simulink model "IEEE24bus"  (R2019b)
settings: Solver=VariableStepAuto  StartTime=0.0  StopTime=100  RelTol=1e-3
values from neighbouring files (symbols this model uses):
  C_b = 1/(w_b*Z_b)    (= 5.01433343075e-06)    [IEEE24_bus.m]
  Exc = [ 011	0	 200	0.02	1.12   0.5   0	0       0       0       0       0 ... (first row only)    [IEEE24_bus.m]
  G_data = [ 011	15.8 138	2.8	0.2     2.7	1.5     0.3     7.5     0.25	0.04	0.85	0.85	0.25	0.12	0 ... (first row only)    [IEEE24_bus.m]
  H011 = 4    [IEEE24_bus.m]
  H012 = 4    [IEEE24_bus.m]
  H013 = 4    [IEEE24_bus.m]
  H021 = 4    [IEEE24_bus.m]
  H022 = 4    [IEEE24_bus.m]
  H023 = 4    [IEEE24_bus.m]
  H024 = 4    [IEEE24_bus.m]
  H025 = 4    [IEEE24_bus.m]
  H026 = 4    [IEEE24_bus.m]
  H131 = 4    [IEEE24_bus.m]
  H132 = 4    [IEEE24_bus.m]
  H133 = 4    [IEEE24_bus.m]
  H134 = 4    [IEEE24_bus.m]
  H135 = 4    [IEEE24_bus.m]
  H151 = 4    [IEEE24_bus.m]
  H152 = 4    [IEEE24_bus.m]
  H153 = 4    [IEEE24_bus.m]
  H154 = 4    [IEEE24_bus.m]
  H161 = 4    [IEEE24_bus.m]
  H181 = 3.25    [IEEE24_bus.m]
  H211 = 4    [IEEE24_bus.m]
  H212 = 4    [IEEE24_bus.m]
  H213 = 4    [IEEE24_bus.m]
  H215 = 4    [IEEE24_bus.m]
  H216 = 4    [IEEE24_bus.m]
  H221 = 3.25    [IEEE24_bus.m]
  H231 = 4    [IEEE24_bus.m]
  H232 = 4    [IEEE24_bus.m]
  H233 = 4    [IEEE24_bus.m]
  H234 = 4    [IEEE24_bus.m]
  H235 = 4    [IEEE24_bus.m]
  L_b = Z_b/w_b    (= 1.40321608159)    [IEEE24_bus.m]
  PSSMODEL = 1    [IEEE24_bus.m]    (also in IEEE24bus_simplified_benchmark.m)
  Z_b = (V_b^2)/S_b    (= 529)    [IEEE24_bus.m]
undefined symbols (not defined in the file or in its folder): D1, Delta
libraries: powerlib x258, sps_avr x33, microgridLibrary x6
(part 5 of 6)

== system IEEE24bus/212 ==
  212 : powerlib/Machines/Synchronous Machine pu Standard  PresetModel=No  MechanicalLoad=Mechanical power Pm  ShowDetailedParameters=on  RotorType=Round  Units=per unit standard parameters  MeasurementBus=off  NominalParameters="[120*1E6  G_data(24,3)*1E3  60]"  Reactances1=[G_data(24,6),G_data(24,8),G_data(24,10),G_data(24,7),G_data(24,12),G_data(24,14),G_data(24,5)]  Reactances2=[G_data(6,6),G_data(6,8),G_data(6,10),G_data(6,7),G_data(6,12),G_data(6,14),G_data(6,5)]  dAxisTimeConstants=Open-circuit  qAxisTimeConstants=Open-circuit  TimeConstants1="[G_data(6,9)  G_data(6,11)  G_data(6,13)  G_data(6,15)]"  TimeConstants2="[G_data(24,9)  G_data(24,11)  G_data(24,13)  G_data(24,15)]"  TimeConstants3="[  5.9  0.033  0.023  ]"  TimeConstants4=[ 8.0, 0.03, 0.3371, 0.0295 ]  TimeConstants5=[ 1.01, 0.053, 0.1 ]  TimeConstants6=[ 1.3201, 0.023, 1.0, 0.07 ]  TimeConstants7="[  1.01  0.053  0.051266  ]"  TimeConstants8=[ 1.3201, 0.0231, 0.3371, 0.0295 ]  StatorResistance=0  Mechanical="[ H212 0  4 ]"  PolePairs=4  InitialConditions=[0 -49.0871 0.832503 0.832503 0.832503 -10.6328 -130.633 109.367 2.39024]  SetSaturation=off  Saturation=[0.6404,0.7127,0.8441,0.9214,0.9956,1.082,1.19,1.316,1.457;0.7,0.7698,0.8872,0.9466,0.9969,1.046,1.1,1.151,1.201]  LoadFlowParameters=[1 3330000000 20000 0 0]  TsPowergui=0  TsBlock=-1  IterativeModel=Forward Euler  IterativeDiscreteModel=Trapezoidal non iterative  BusType=PV  Pref=G_data(24,2)*1e6  Qref=0  Qmin=-inf  Qmax=inf  PLF=0  QLF=0
      settings: SourceProductName=Simscape Power Systems
  AC4A Excitation System 212 : sps_avr/AC4A Excitation System  Tr=Exc(24,2)  KaTa="[Exc(24,3)   Exc(24,4)]"  VIminmax=[-10 10]  VRminmax=[-4.53 5.64]  TbTc="[Exc(24,5)  Exc(24,6)]"  Kc=0  v0=[1 2.3902]  TsBlock=0
      settings: SourceProductName=Simscape Power Systems  SourceProductBaseCode=PS
  Bus Selector1 : BusSelector  OutputSignals="Mechanical.Rotor speed  wm  (pu),Output active power   Peo (pu),Mechanical.Rotor speed deviation  dw (pu),Mechanical.Rotor angle deviation  d_theta (rad),Mechanical.Rotor mechanical angle  theta (deg),dq0 components.Stator voltage  vd (pu),dq0 components.Stator voltage  vq (pu),dq0 components.Field current  ifd (pu),Output reactive power  Qeo (pu)"
  Complex to Magnitude-Angle : ComplexToMagnitudeAngle  Output=Magnitude
  "Delta Pa PSS 212 " : powerlib/Machines/Generic Power System Stabilizer  Tsensor=15e-3  K=2.5*1.25  Twashout=1  Tleadlag1=[60e-3 1]  Tleadlag2=[0 0]  VSlimits=[-0.15 0.15]  Vinit=0  Plot_On=off  MagdB_On=on  FreqRange=logspace(-2,2,500)
      settings: SourceProductName=Simscape Power Systems  SourceProductBaseCode=PS
  "Delta w PSS (Kundur) 212 " : powerlib/Machines/Generic Power System Stabilizer  Tsensor=15e-3  K=30  Twashout=10  Tleadlag1=[50e-3 20e-3]  Tleadlag2=[3 5.4]  VSlimits=[-0.15 0.15]  Vinit=0  Plot_On=off  MagdB_On=on  FreqRange=logspace(-2,2,500)
      settings: SourceProductName=Simscape Power Systems  SourceProductBaseCode=PS
  MB-PSS  212 : powerlib/Machines/Multi-Band Power System Stabilizer  OperationMode=Simplified settings  Kg=1  GL=[0.1 10]  GI="[1  10]"  GH="[13  120]"  GLd=[66 66 9.4]  TcLF=[1.667 2 0 0 0 0 2 2.4 0 0 0 0 1 1]  GId=[66 66 47.6]  TcIF=[1 1 0.25 0.3 0 0 1 1 0.3 0.36 0 0 0 0]  GHd=[66 66 233]  TcHF="[0.01 0.012 0 0 0 0  0.012 0.0144 0 0 0 0 1 1]"  LIM=[.075 .15 .15 .15]  Plot_On=off  MagdB_On=off  FreqRange=logspace(-2,2,500)
      settings: SourceProductName=Simscape Power Systems  SourceProductBaseCode=PS
  Multiport Switch1 : MultiPortSwitch  Inputs=4  InputSameDT=on
  PSS model3 : Constant  Value=0
  PSS model4 : Constant
  Pref : Constant
  Real-Imag to Complex : RealImagToComplex
  STG 212 : powerlib/Machines/Steam Turbine and Governor  gentype=Tandem-compound (single mass)  reg1="[ 1  0.05    0 ]"  reg2="[ 0.001  0.15 ]"  reg3="[ -0.1  0.1  0  4.496 ]"  N=3600  turb1="[ 0  10   3.3   0.5   ]"  turb2="[   0   0.36    0.36   0.28   ]"  HA="[ 0.046  1.430  1.465   0.192 ]"  KA="[ 90.44  53.88  64.59   62.94  ]"  DA="[ 0.0115  0.3575  0.3663   0.0137  ]"  ini1=0.451  ini2=[0.779316,-31.4247]
      settings: SourceProductName=Simscape Power Systems  SourceProductBaseCode=PS
  Sum2 : Sum  SaturateOnIntegerOverflow=on  InputSameDT=on  OutDataTypeStr=Inherit: Same as first input
  Sum3 : Sum  Inputs=-+  SaturateOnIntegerOverflow=on  InputSameDT=on  OutDataTypeStr=Inherit: Same as first input
  Terminator1 : Terminator
  Terminator2 : Terminator
  Terminator3 : Terminator
  Vref21 : Constant
  wref : Constant
  A : PMIOPort  Side=Left
  B : PMIOPort  Port=2  Side=Left
  C : PMIOPort  Port=3  Side=Left
  tag scope: EFD212=global, Pa212=global, Pe212=global, Pm212=global, Q212=global, Vt212=global, d_theta212=global, pss212=global, theta212=global, w212=global
  wires:
  Bus Selector1/7 -> Real-Imag to Complex/2  "<Stator voltage  vq (pu)>"
  Bus Selector1/6 -> Real-Imag to Complex/1  "<Stator voltage  vd (pu)>"
  wref/1 -> STG 212/1
  Vref21/1 -> AC4A Excitation System 212/1
  Bus Selector1/4 -> [d_theta212], STG 212/4  "<Rotor angle deviation  d_theta (rad)>"
  212/1 -> Bus Selector1/1, [M212]
  Bus Selector1/1 -> [w212], STG 212/3  "<Rotor speed  wm  (pu)>"
  Bus Selector1/3 -> "Delta w PSS (Kundur) 212 "/1, MB-PSS  212/1  "<Rotor speed deviation  dw (pu)>"
  Real-Imag to Complex/1 -> Complex to Magnitude-Angle/1
  Complex to Magnitude-Angle/1 -> AC4A Excitation System 212/2, [Vt212]
  AC4A Excitation System 212/1 -> 212/2, [EFD212]
  Multiport Switch1/1 -> AC4A Excitation System 212/4, [pss212]
  Bus Selector1/5 -> [theta212]  "<Rotor mechanical angle  theta (deg)>"
  Bus Selector1/2 -> [Pe212]  "<Output active power   Peo (pu)>"
  Bus Selector1/8 -> AC4A Excitation System 212/3  "<Field current  ifd (pu)>"
  STG 212/4 -> [Pm212], 212/1
  Pref/1 -> STG 212/2
  Bus Selector1/9 -> [Q212]  "<Output reactive power  Qeo (pu)>"
  PSS model4/1 -> Sum2/2
  Sum2/1 -> Multiport Switch1/1
  [PSSmodel] -> Sum2/1
  PSS model3/1 -> Multiport Switch1/2
  Sum3/1 -> [Pa212], "Delta Pa PSS 212 "/1  "Pm-Pe"
  "Delta Pa PSS 212 "/1 -> Multiport Switch1/5
  "Delta w PSS (Kundur) 212 "/1 -> Multiport Switch1/4
  [Pm212] -> Sum3/2
  [Pe212] -> Sum3/1
  MB-PSS  212/1 -> Multiport Switch1/3
  STG 212/1 -> Terminator3/1
  STG 212/2 -> Terminator1/1
  STG 212/3 -> Terminator2/1
  connections:
  212/RConn1 -- A/RConn1
  212/RConn2 -- B/RConn1
  212/RConn3 -- C/RConn1

== system IEEE24bus/213 ==
  213 : powerlib/Machines/Synchronous Machine pu Standard  PresetModel=No  MechanicalLoad=Mechanical power Pm  ShowDetailedParameters=on  RotorType=Round  Units=per unit standard parameters  MeasurementBus=off  NominalParameters="[120*1E6  (130+G_data(25,3))*1E3  60]"  Reactances1=[G_data(25,6),G_data(25,8),G_data(25,10),G_data(25,7),G_data(25,12),G_data(25,14),G_data(25,5)]  Reactances2=[G_data(6,6),G_data(6,8),G_data(6,10),G_data(6,7),G_data(6,12),G_data(6,14),G_data(6,5)]  dAxisTimeConstants=Open-circuit  qAxisTimeConstants=Open-circuit  TimeConstants1="[G_data(6,9)  G_data(6,11)  G_data(6,13)  G_data(6,15)]"  TimeConstants2="[G_data(25,9)  G_data(25,11)  G_data(25,13)  G_data(25,15)]"  TimeConstants3="[  5.9  0.033  0.023  ]"  TimeConstants4=[ 8.0, 0.03, 0.3371, 0.0295 ]  TimeConstants5=[ 1.01, 0.053, 0.1 ]  TimeConstants6=[ 1.3201, 0.023, 1.0, 0.07 ]  TimeConstants7="[  1.01  0.053  0.051266  ]"  TimeConstants8=[ 1.3201, 0.0231, 0.3371, 0.0295 ]  StatorResistance=0  Mechanical="[ H213 0  4 ]"  PolePairs=4  InitialConditions=[0 -49.0871 0.832503 0.832503 0.832503 -10.6328 -130.633 109.367 2.39024]  SetSaturation=off  Saturation=[0.6404,0.7127,0.8441,0.9214,0.9956,1.082,1.19,1.316,1.457;0.7,0.7698,0.8872,0.9466,0.9969,1.046,1.1,1.151,1.201]  LoadFlowParameters=[1 3330000000 20000 0 0]  TsPowergui=0  TsBlock=-1  IterativeModel=Forward Euler  IterativeDiscreteModel=Trapezoidal non iterative  BusType=PV  Pref=G_data(25,2)*1e6  Qref=0  Qmin=-inf  Qmax=inf  PLF=0  QLF=0
      settings: SourceProductName=Simscape Power Systems
  AC4A Excitation System 21 : sps_avr/AC4A Excitation System  Tr=Exc(25,2)  KaTa="[Exc(25,3)   Exc(25,4)]"  VIminmax=[-10 10]  VRminmax=[-4.53 5.64]  TbTc="[Exc(25,5)  Exc(25,6)]"  Kc=0  v0=[1 2.3902]  TsBlock=0
      settings: SourceProductName=Simscape Power Systems  SourceProductBaseCode=PS
  Bus Selector1 : BusSelector  OutputSignals="Mechanical.Rotor speed  wm  (pu),Output active power   Peo (pu),Mechanical.Rotor speed deviation  dw (pu),Mechanical.Rotor angle deviation  d_theta (rad),Mechanical.Rotor mechanical angle  theta (deg),dq0 components.Stator voltage  vd (pu),dq0 components.Stator voltage  vq (pu),dq0 components.Field current  ifd (pu),Output reactive power  Qeo (pu)"
  Complex to Magnitude-Angle : ComplexToMagnitudeAngle  Output=Magnitude
  "Delta Pa PSS 213 " : powerlib/Machines/Generic Power System Stabilizer  Tsensor=15e-3  K=2.5*1.25  Twashout=1  Tleadlag1=[60e-3 1]  Tleadlag2=[0 0]  VSlimits=[-0.15 0.15]  Vinit=0  Plot_On=off  MagdB_On=on  FreqRange=logspace(-2,2,500)
      settings: SourceProductName=Simscape Power Systems  SourceProductBaseCode=PS
  "Delta w PSS (Kundur) 213 " : powerlib/Machines/Generic Power System Stabilizer  Tsensor=15e-3  K=30  Twashout=10  Tleadlag1=[50e-3 20e-3]  Tleadlag2=[3 5.4]  VSlimits=[-0.15 0.15]  Vinit=0  Plot_On=off  MagdB_On=on  FreqRange=logspace(-2,2,500)
      settings: SourceProductName=Simscape Power Systems  SourceProductBaseCode=PS
  MB-PSS  213 : powerlib/Machines/Multi-Band Power System Stabilizer  OperationMode=Simplified settings  Kg=1  GL=[0.1 10]  GI="[1  10]"  GH="[13  120]"  GLd=[66 66 9.4]  TcLF=[1.667 2 0 0 0 0 2 2.4 0 0 0 0 1 1]  GId=[66 66 47.6]  TcIF=[1 1 0.25 0.3 0 0 1 1 0.3 0.36 0 0 0 0]  GHd=[66 66 233]  TcHF="[0.01 0.012 0 0 0 0  0.012 0.0144 0 0 0 0 1 1]"  LIM=[.075 .15 .15 .15]  Plot_On=off  MagdB_On=off  FreqRange=logspace(-2,2,500)
      settings: SourceProductName=Simscape Power Systems  SourceProductBaseCode=PS
  Multiport Switch1 : MultiPortSwitch  Inputs=4  InputSameDT=on
  PSS model3 : Constant  Value=0
  PSS model4 : Constant
  Pref : Constant
  Real-Imag to Complex : RealImagToComplex
  STG 213 : powerlib/Machines/Steam Turbine and Governor  gentype=Tandem-compound (single mass)  reg1="[ 1  0.05    0 ]"  reg2="[ 0.001  0.15 ]"  reg3="[ -0.1  0.1  0  4.496 ]"  N=3600  turb1="[ 0  10   3.3   0.5   ]"  turb2="[   0   0.36    0.36   0.28   ]"  HA="[ 0.046  1.430  1.465   0.192 ]"  KA="[ 90.44  53.88  64.59   62.94  ]"  DA="[ 0.0115  0.3575  0.3663   0.0137  ]"  ini1=0.451  ini2=[0.779316,-31.4247]
      settings: SourceProductName=Simscape Power Systems  SourceProductBaseCode=PS
  Sum2 : Sum  SaturateOnIntegerOverflow=on  InputSameDT=on  OutDataTypeStr=Inherit: Same as first input
  Sum3 : Sum  Inputs=-+  SaturateOnIntegerOverflow=on  InputSameDT=on  OutDataTypeStr=Inherit: Same as first input
  Terminator1 : Terminator
  Terminator2 : Terminator
  Terminator3 : Terminator
  Vref21 : Constant
  wref : Constant
  A : PMIOPort  Side=Left
  B : PMIOPort  Port=2  Side=Left
  C : PMIOPort  Port=3  Side=Left
  tag scope: EFD213=global, Pa213=global, Pe213=global, Pm213=global, Q213=global, Vt213=global, d_theta213=global, pss213=global, theta213=global, w213=global
  wires:
  Bus Selector1/7 -> Real-Imag to Complex/2  "<Stator voltage  vq (pu)>"
  Bus Selector1/6 -> Real-Imag to Complex/1  "<Stator voltage  vd (pu)>"
  wref/1 -> STG 213/1
  Vref21/1 -> AC4A Excitation System 21/1
  Bus Selector1/4 -> [d_theta213], STG 213/4  "<Rotor angle deviation  d_theta (rad)>"
  213/1 -> Bus Selector1/1, [M213]
  Bus Selector1/1 -> [w213], STG 213/3  "<Rotor speed  wm  (pu)>"
  Bus Selector1/3 -> "Delta w PSS (Kundur) 213 "/1, MB-PSS  213/1  "<Rotor speed deviation  dw (pu)>"
  Real-Imag to Complex/1 -> Complex to Magnitude-Angle/1
  Complex to Magnitude-Angle/1 -> AC4A Excitation System 21/2, [Vt213]
  AC4A Excitation System 21/1 -> 213/2, [EFD213]
  Multiport Switch1/1 -> AC4A Excitation System 21/4, [pss213]
  Bus Selector1/5 -> [theta213]  "<Rotor mechanical angle  theta (deg)>"
  Bus Selector1/2 -> [Pe213]  "<Output active power   Peo (pu)>"
  Bus Selector1/8 -> AC4A Excitation System 21/3  "<Field current  ifd (pu)>"
  STG 213/4 -> [Pm213], 213/1
  Pref/1 -> STG 213/2
  Bus Selector1/9 -> [Q213]  "<Output reactive power  Qeo (pu)>"
  PSS model4/1 -> Sum2/2
  Sum2/1 -> Multiport Switch1/1
  [PSSmodel] -> Sum2/1
  PSS model3/1 -> Multiport Switch1/2
  Sum3/1 -> [Pa213], "Delta Pa PSS 213 "/1  "Pm-Pe"
  "Delta Pa PSS 213 "/1 -> Multiport Switch1/5
  "Delta w PSS (Kundur) 213 "/1 -> Multiport Switch1/4
  [Pm213] -> Sum3/2
  [Pe213] -> Sum3/1
  MB-PSS  213/1 -> Multiport Switch1/3
  STG 213/1 -> Terminator3/1
  STG 213/2 -> Terminator1/1
  STG 213/3 -> Terminator2/1
  connections:
  213/RConn1 -- A/RConn1
  213/RConn2 -- B/RConn1
  213/RConn3 -- C/RConn1

== system IEEE24bus/214 ==
  214 : powerlib/Machines/Synchronous Machine pu Standard  PresetModel=No  MechanicalLoad=Mechanical power Pm  ShowDetailedParameters=on  RotorType=Round  Units=per unit standard parameters  MeasurementBus=off  NominalParameters="[120*1E6  G_data(26,3)*1E3  60]"  Reactances1=[G_data(26,6),G_data(26,8),G_data(26,10),G_data(26,7),G_data(26,12),G_data(26,14),G_data(26,5)]  Reactances2=[G_data(6,6),G_data(6,8),G_data(6,10),G_data(6,7),G_data(6,12),G_data(6,14),G_data(6,5)]  dAxisTimeConstants=Open-circuit  qAxisTimeConstants=Open-circuit  TimeConstants1="[G_data(6,9)  G_data(6,11)  G_data(6,13)  G_data(6,15)]"  TimeConstants2="[G_data(26,9)  G_data(26,11)  G_data(26,13)  G_data(26,15)]"  TimeConstants3="[  5.9  0.033  0.023  ]"  TimeConstants4=[ 8.0, 0.03, 0.3371, 0.0295 ]  TimeConstants5=[ 1.01, 0.053, 0.1 ]  TimeConstants6=[ 1.3201, 0.023, 1.0, 0.07 ]  TimeConstants7="[  1.01  0.053  0.051266  ]"  TimeConstants8=[ 1.3201, 0.0231, 0.3371, 0.0295 ]  StatorResistance=0  Mechanical="[ H216 0  4 ]"  PolePairs=4  InitialConditions=[0 -49.0871 0.832503 0.832503 0.832503 -10.6328 -130.633 109.367 2.39024]  SetSaturation=off  Saturation=[0.6404,0.7127,0.8441,0.9214,0.9956,1.082,1.19,1.316,1.457;0.7,0.7698,0.8872,0.9466,0.9969,1.046,1.1,1.151,1.201]  LoadFlowParameters=[1 3330000000 20000 0 0]  TsPowergui=0  TsBlock=-1  IterativeModel=Forward Euler  IterativeDiscreteModel=Trapezoidal non iterative  BusType=PV  Pref=G_data(26,2)*1e6  Qref=0  Qmin=-inf  Qmax=inf  PLF=0  QLF=0
      settings: SourceProductName=Simscape Power Systems
  AC4A Excitation System 214 : sps_avr/AC4A Excitation System  Tr=Exc(26,2)  KaTa="[Exc(26,3)   Exc(26,4)]"  VIminmax=[-10 10]  VRminmax=[-4.53 5.64]  TbTc="[Exc(26,5)  Exc(26,6)]"  Kc=0  v0=[1 2.3902]  TsBlock=0
      settings: SourceProductName=Simscape Power Systems  SourceProductBaseCode=PS
  Bus Selector1 : BusSelector  OutputSignals="Mechanical.Rotor speed  wm  (pu),Output active power   Peo (pu),Mechanical.Rotor speed deviation  dw (pu),Mechanical.Rotor angle deviation  d_theta (rad),Mechanical.Rotor mechanical angle  theta (deg),dq0 components.Stator voltage  vd (pu),dq0 components.Stator voltage  vq (pu),dq0 components.Field current  ifd (pu),Output reactive power  Qeo (pu)"
  Complex to Magnitude-Angle : ComplexToMagnitudeAngle  Output=Magnitude
  "Delta Pa PSS 214 " : powerlib/Machines/Generic Power System Stabilizer  Tsensor=15e-3  K=2.5*1.25  Twashout=1  Tleadlag1=[60e-3 1]  Tleadlag2=[0 0]  VSlimits=[-0.15 0.15]  Vinit=0  Plot_On=off  MagdB_On=on  FreqRange=logspace(-2,2,500)
      settings: SourceProductName=Simscape Power Systems  SourceProductBaseCode=PS
  "Delta w PSS (Kundur) 214 " : powerlib/Machines/Generic Power System Stabilizer  Tsensor=15e-3  K=30  Twashout=10  Tleadlag1=[50e-3 20e-3]  Tleadlag2=[3 5.4]  VSlimits=[-0.15 0.15]  Vinit=0  Plot_On=off  MagdB_On=on  FreqRange=logspace(-2,2,500)
      settings: SourceProductName=Simscape Power Systems  SourceProductBaseCode=PS
  MB-PSS  214 : powerlib/Machines/Multi-Band Power System Stabilizer  OperationMode=Simplified settings  Kg=1  GL=[0.1 10]  GI="[1  10]"  GH="[13  120]"  GLd=[66 66 9.4]  TcLF=[1.667 2 0 0 0 0 2 2.4 0 0 0 0 1 1]  GId=[66 66 47.6]  TcIF=[1 1 0.25 0.3 0 0 1 1 0.3 0.36 0 0 0 0]  GHd=[66 66 233]  TcHF="[0.01 0.012 0 0 0 0  0.012 0.0144 0 0 0 0 1 1]"  LIM=[.075 .15 .15 .15]  Plot_On=off  MagdB_On=off  FreqRange=logspace(-2,2,500)
      settings: SourceProductName=Simscape Power Systems  SourceProductBaseCode=PS
  Multiport Switch1 : MultiPortSwitch  Inputs=4  InputSameDT=on
  PSS model3 : Constant  Value=0
  PSS model4 : Constant
  Pref : Constant
  Real-Imag to Complex : RealImagToComplex
  STG 214 : powerlib/Machines/Steam Turbine and Governor  gentype=Tandem-compound (single mass)  reg1="[ 1  0.05    0 ]"  reg2="[ 0.001  0.15 ]"  reg3="[ -0.1  0.1  0  4.496 ]"  N=3600  turb1="[ 0  10   3.3   0.5   ]"  turb2="[   0   0.36    0.36   0.28   ]"  HA="[ 0.046  1.430  1.465   0.192 ]"  KA="[ 90.44  53.88  64.59   62.94  ]"  DA="[ 0.0115  0.3575  0.3663   0.0137  ]"  ini1=0.451  ini2=[0.779316,-31.4247]
      settings: SourceProductName=Simscape Power Systems  SourceProductBaseCode=PS
  Sum2 : Sum  SaturateOnIntegerOverflow=on  InputSameDT=on  OutDataTypeStr=Inherit: Same as first input
  Sum3 : Sum  Inputs=-+  SaturateOnIntegerOverflow=on  InputSameDT=on  OutDataTypeStr=Inherit: Same as first input
  Terminator1 : Terminator
  Terminator2 : Terminator
  Terminator3 : Terminator
  Vref21 : Constant
  wref : Constant
  A : PMIOPort  Side=Left
  B : PMIOPort  Port=2  Side=Left
  C : PMIOPort  Port=3  Side=Left
  tag scope: EFD214=global, Pa214=global, Pe214=global, Pm214=global, Q214=global, Vt214=global, d_theta214=global, pss214=global, theta214=global, w214=global
  wires:
  Bus Selector1/7 -> Real-Imag to Complex/2  "<Stator voltage  vq (pu)>"
  Bus Selector1/6 -> Real-Imag to Complex/1  "<Stator voltage  vd (pu)>"
  wref/1 -> STG 214/1
  Vref21/1 -> AC4A Excitation System 214/1
  Bus Selector1/4 -> [d_theta214], STG 214/4  "<Rotor angle deviation  d_theta (rad)>"
  214/1 -> Bus Selector1/1, [M214]
  Bus Selector1/1 -> [w214], STG 214/3  "<Rotor speed  wm  (pu)>"
  Bus Selector1/3 -> "Delta w PSS (Kundur) 214 "/1, MB-PSS  214/1  "<Rotor speed deviation  dw (pu)>"
  Real-Imag to Complex/1 -> Complex to Magnitude-Angle/1
  Complex to Magnitude-Angle/1 -> AC4A Excitation System 214/2, [Vt214]
  AC4A Excitation System 214/1 -> 214/2, [EFD214]
  Multiport Switch1/1 -> AC4A Excitation System 214/4, [pss214]
  Bus Selector1/5 -> [theta214]  "<Rotor mechanical angle  theta (deg)>"
  Bus Selector1/2 -> [Pe214]  "<Output active power   Peo (pu)>"
  Bus Selector1/8 -> AC4A Excitation System 214/3  "<Field current  ifd (pu)>"
  STG 214/4 -> [Pm214], 214/1
  Pref/1 -> STG 214/2
  Bus Selector1/9 -> [Q214]  "<Output reactive power  Qeo (pu)>"
  PSS model4/1 -> Sum2/2
  Sum2/1 -> Multiport Switch1/1
  [PSSmodel] -> Sum2/1
  PSS model3/1 -> Multiport Switch1/2
  Sum3/1 -> [Pa214], "Delta Pa PSS 214 "/1  "Pm-Pe"
  "Delta Pa PSS 214 "/1 -> Multiport Switch1/5
  "Delta w PSS (Kundur) 214 "/1 -> Multiport Switch1/4
  [Pm21] -> Sum3/2
  [Pe21] -> Sum3/1
  MB-PSS  214/1 -> Multiport Switch1/3
  STG 214/1 -> Terminator3/1
  STG 214/2 -> Terminator1/1
  STG 214/3 -> Terminator2/1
  connections:
  214/RConn1 -- A/RConn1
  214/RConn2 -- B/RConn1
  214/RConn3 -- C/RConn1

== system IEEE24bus/215 ==
  215 : powerlib/Machines/Synchronous Machine pu Standard  PresetModel=No  MechanicalLoad=Mechanical power Pm  ShowDetailedParameters=on  RotorType=Round  Units=per unit standard parameters  MeasurementBus=off  NominalParameters="[G_data(27,2)*1E6  G_data(27,3)*1E3  60]"  Reactances1=[G_data(27,6),G_data(27,8),G_data(27,10),G_data(27,7),G_data(27,12),G_data(27,14),G_data(27,5)]  Reactances2=[G_data(6,6),G_data(6,8),G_data(6,10),G_data(6,7),G_data(6,12),G_data(6,14),G_data(6,5)]  dAxisTimeConstants=Open-circuit  qAxisTimeConstants=Open-circuit  TimeConstants1="[G_data(6,9)  G_data(6,11)  G_data(6,13)  G_data(6,15)]"  TimeConstants2="[G_data(27,9)  G_data(27,11)  G_data(27,13)  G_data(27,15)]"  TimeConstants3="[  5.9  0.033  0.023  ]"  TimeConstants4=[ 8.0, 0.03, 0.3371, 0.0295 ]  TimeConstants5=[ 1.01, 0.053, 0.1 ]  TimeConstants6=[ 1.3201, 0.023, 1.0, 0.07 ]  TimeConstants7="[  1.01  0.053  0.051266  ]"  TimeConstants8=[ 1.3201, 0.0231, 0.3371, 0.0295 ]  StatorResistance=0  Mechanical="[ H215 0  4 ]"  PolePairs=4  InitialConditions=[0 -49.0871 0.832503 0.832503 0.832503 -10.6328 -130.633 109.367 2.39024]  SetSaturation=off  Saturation=[0.6404,0.7127,0.8441,0.9214,0.9956,1.082,1.19,1.316,1.457;0.7,0.7698,0.8872,0.9466,0.9969,1.046,1.1,1.151,1.201]  LoadFlowParameters=[1 3330000000 20000 0 0]  TsPowergui=0  TsBlock=-1  IterativeModel=Forward Euler  IterativeDiscreteModel=Trapezoidal non iterative  BusType=PV  Pref=G_data(27,2)*1e6  Qref=0  Qmin=-inf  Qmax=inf  PLF=0  QLF=0
      settings: SourceProductName=Simscape Power Systems
  AC4A Excitation System 215 : sps_avr/AC4A Excitation System  Tr=Exc(27,2)  KaTa="[Exc(27,3)   Exc(27,4)]"  VIminmax=[-10 10]  VRminmax=[-4.53 5.64]  TbTc="[Exc(27,5)  Exc(27,6)]"  Kc=0  v0=[1 2.3902]  TsBlock=0
      settings: SourceProductName=Simscape Power Systems  SourceProductBaseCode=PS
  Bus Selector1 : BusSelector  OutputSignals="Mechanical.Rotor speed  wm  (pu),Output active power   Peo (pu),Mechanical.Rotor speed deviation  dw (pu),Mechanical.Rotor angle deviation  d_theta (rad),Mechanical.Rotor mechanical angle  theta (deg),dq0 components.Stator voltage  vd (pu),dq0 components.Stator voltage  vq (pu),dq0 components.Field current  ifd (pu),Output reactive power  Qeo (pu)"
  Complex to Magnitude-Angle : ComplexToMagnitudeAngle  Output=Magnitude
  Delta Pa PSS 215 : powerlib/Machines/Generic Power System Stabilizer  Tsensor=15e-3  K=2.5*1.25  Twashout=1  Tleadlag1=[60e-3 1]  Tleadlag2=[0 0]  VSlimits=[-0.15 0.15]  Vinit=0  Plot_On=off  MagdB_On=on  FreqRange=logspace(-2,2,500)
      settings: SourceProductName=Simscape Power Systems  SourceProductBaseCode=PS
  "Delta w PSS (Kundur) 215 " : powerlib/Machines/Generic Power System Stabilizer  Tsensor=15e-3  K=30  Twashout=10  Tleadlag1=[50e-3 20e-3]  Tleadlag2=[3 5.4]  VSlimits=[-0.15 0.15]  Vinit=0  Plot_On=off  MagdB_On=on  FreqRange=logspace(-2,2,500)
      settings: SourceProductName=Simscape Power Systems  SourceProductBaseCode=PS
  MB-PSS  215 : powerlib/Machines/Multi-Band Power System Stabilizer  OperationMode=Simplified settings  Kg=1  GL=[0.1 10]  GI="[1  10]"  GH="[13  120]"  GLd=[66 66 9.4]  TcLF=[1.667 2 0 0 0 0 2 2.4 0 0 0 0 1 1]  GId=[66 66 47.6]  TcIF=[1 1 0.25 0.3 0 0 1 1 0.3 0.36 0 0 0 0]  GHd=[66 66 233]  TcHF="[0.01 0.012 0 0 0 0  0.012 0.0144 0 0 0 0 1 1]"  LIM=[.075 .15 .15 .15]  Plot_On=off  MagdB_On=off  FreqRange=logspace(-2,2,500)
      settings: SourceProductName=Simscape Power Systems  SourceProductBaseCode=PS
  Multiport Switch1 : MultiPortSwitch  Inputs=4  InputSameDT=on
  PSS model3 : Constant  Value=0
  PSS model4 : Constant
  Pref : Constant
  Real-Imag to Complex : RealImagToComplex
  STG 215 : powerlib/Machines/Steam Turbine and Governor  gentype=Tandem-compound (single mass)  reg1="[ 1  0.05    0 ]"  reg2="[ 0.001  0.15 ]"  reg3="[ -0.1  0.1  0  4.496 ]"  N=3600  turb1="[ 0  10   3.3   0.5   ]"  turb2="[   0   0.36    0.36   0.28   ]"  HA="[ 0.046  1.430  1.465   0.192 ]"  KA="[ 90.44  53.88  64.59   62.94  ]"  DA="[ 0.0115  0.3575  0.3663   0.0137  ]"  ini1=0.9  ini2=[0.779316,-31.4247]
      settings: SourceProductName=Simscape Power Systems  SourceProductBaseCode=PS
  Sum2 : Sum  SaturateOnIntegerOverflow=on  InputSameDT=on  OutDataTypeStr=Inherit: Same as first input
  Sum3 : Sum  Inputs=-+  SaturateOnIntegerOverflow=on  InputSameDT=on  OutDataTypeStr=Inherit: Same as first input
  Terminator1 : Terminator
  Terminator2 : Terminator
  Terminator3 : Terminator
  Vref21 : Constant
  wref : Constant
  A : PMIOPort  Side=Left
  B : PMIOPort  Port=2  Side=Left
  C : PMIOPort  Port=3  Side=Left
  tag scope: EFD215=global, Pa215=global, Pe215=global, Pm215=global, Q215=global, Vt215=global, d_theta215=global, pss215=global, theta215=global, w215=global
  wires:
  Bus Selector1/7 -> Real-Imag to Complex/2  "<Stator voltage  vq (pu)>"
  Bus Selector1/6 -> Real-Imag to Complex/1  "<Stator voltage  vd (pu)>"
  wref/1 -> STG 215/1
  Vref21/1 -> AC4A Excitation System 215/1
  Bus Selector1/4 -> [d_theta215], STG 215/4  "<Rotor angle deviation  d_theta (rad)>"
  215/1 -> Bus Selector1/1, [M215]
  Bus Selector1/1 -> [w215], STG 215/3  "<Rotor speed  wm  (pu)>"
  Bus Selector1/3 -> "Delta w PSS (Kundur) 215 "/1, MB-PSS  215/1  "<Rotor speed deviation  dw (pu)>"
  Real-Imag to Complex/1 -> Complex to Magnitude-Angle/1
  Complex to Magnitude-Angle/1 -> AC4A Excitation System 215/2, [Vt215]
  AC4A Excitation System 215/1 -> 215/2, [EFD215]
  Multiport Switch1/1 -> AC4A Excitation System 215/4, [pss215]
  Bus Selector1/5 -> [theta215]  "<Rotor mechanical angle  theta (deg)>"
  Bus Selector1/2 -> [Pe215]  "<Output active power   Peo (pu)>"
  Bus Selector1/8 -> AC4A Excitation System 215/3  "<Field current  ifd (pu)>"
  STG 215/4 -> [Pm215], 215/1
  Pref/1 -> STG 215/2
  Bus Selector1/9 -> [Q215]  "<Output reactive power  Qeo (pu)>"
  PSS model4/1 -> Sum2/2
  Sum2/1 -> Multiport Switch1/1
  [PSSmodel] -> Sum2/1
  PSS model3/1 -> Multiport Switch1/2
  Sum3/1 -> [Pa215], Delta Pa PSS 215/1  "Pm-Pe"
  Delta Pa PSS 215/1 -> Multiport Switch1/5
  "Delta w PSS (Kundur) 215 "/1 -> Multiport Switch1/4
  [Pm215] -> Sum3/2
  [Pe215] -> Sum3/1
  MB-PSS  215/1 -> Multiport Switch1/3
  STG 215/1 -> Terminator3/1
  STG 215/2 -> Terminator1/1
  STG 215/3 -> Terminator2/1
  connections:
  215/RConn1 -- A/RConn1
  215/RConn2 -- B/RConn1
  215/RConn3 -- C/RConn1

== system IEEE24bus/216 ==
  216 : powerlib/Machines/Synchronous Machine pu Standard  PresetModel=No  MechanicalLoad=Mechanical power Pm  ShowDetailedParameters=on  RotorType=Round  Units=per unit standard parameters  MeasurementBus=off  NominalParameters="[G_data(28,2)*1E6  G_data(28,3)*1E3  60]"  Reactances1=[G_data(28,6),G_data(28,8),G_data(28,10),G_data(28,7),G_data(28,12),G_data(28,14),G_data(28,5)]  Reactances2=[G_data(6,6),G_data(6,8),G_data(6,10),G_data(6,7),G_data(6,12),G_data(6,14),G_data(6,5)]  dAxisTimeConstants=Open-circuit  qAxisTimeConstants=Open-circuit  TimeConstants1="[G_data(6,9)  G_data(6,11)  G_data(6,13)  G_data(6,15)]"  TimeConstants2="[G_data(28,9)  G_data(28,11)  G_data(28,13)  G_data(28,15)]"  TimeConstants3="[  5.9  0.033  0.023  ]"  TimeConstants4=[ 8.0, 0.03, 0.3371, 0.0295 ]  TimeConstants5=[ 1.01, 0.053, 0.1 ]  TimeConstants6=[ 1.3201, 0.023, 1.0, 0.07 ]  TimeConstants7="[  1.01  0.053  0.051266  ]"  TimeConstants8=[ 1.3201, 0.0231, 0.3371, 0.0295 ]  StatorResistance=0  Mechanical="[ H216 0  4 ]"  PolePairs=4  InitialConditions=[0 -49.0871 0.832503 0.832503 0.832503 -10.6328 -130.633 109.367 2.39024]  SetSaturation=off  Saturation=[0.6404,0.7127,0.8441,0.9214,0.9956,1.082,1.19,1.316,1.457;0.7,0.7698,0.8872,0.9466,0.9969,1.046,1.1,1.151,1.201]  LoadFlowParameters=[1 3330000000 20000 0 0]  TsPowergui=0  TsBlock=-1  IterativeModel=Forward Euler  IterativeDiscreteModel=Trapezoidal non iterative  BusType=PV  Pref=G_data(28,2)*1e6  Qref=0  Qmin=-inf  Qmax=inf  PLF=0  QLF=0
      settings: SourceProductName=Simscape Power Systems
  AC4A Excitation System 216 : sps_avr/AC4A Excitation System  Tr=Exc(28,2)  KaTa="[Exc(28,3)   Exc(28,4)]"  VIminmax=[-10 10]  VRminmax=[-4.53 5.64]  TbTc="[Exc(28,5)  Exc(28,6)]"  Kc=0  v0=[1 2.3902]  TsBlock=0
      settings: SourceProductName=Simscape Power Systems  SourceProductBaseCode=PS
  Bus Selector1 : BusSelector  OutputSignals="Mechanical.Rotor speed  wm  (pu),Output active power   Peo (pu),Mechanical.Rotor speed deviation  dw (pu),Mechanical.Rotor angle deviation  d_theta (rad),Mechanical.Rotor mechanical angle  theta (deg),dq0 components.Stator voltage  vd (pu),dq0 components.Stator voltage  vq (pu),dq0 components.Field current  ifd (pu),Output reactive power  Qeo (pu)"
  Complex to Magnitude-Angle : ComplexToMagnitudeAngle  Output=Magnitude
  "Delta Pa PSS 216 " : powerlib/Machines/Generic Power System Stabilizer  Tsensor=15e-3  K=2.5*1.25  Twashout=1  Tleadlag1=[60e-3 1]  Tleadlag2=[0 0]  VSlimits=[-0.15 0.15]  Vinit=0  Plot_On=off  MagdB_On=on  FreqRange=logspace(-2,2,500)
      settings: SourceProductName=Simscape Power Systems  SourceProductBaseCode=PS
  "Delta w PSS (Kundur) 216 " : powerlib/Machines/Generic Power System Stabilizer  Tsensor=15e-3  K=30  Twashout=10  Tleadlag1=[50e-3 20e-3]  Tleadlag2=[3 5.4]  VSlimits=[-0.15 0.15]  Vinit=0  Plot_On=off  MagdB_On=on  FreqRange=logspace(-2,2,500)
      settings: SourceProductName=Simscape Power Systems  SourceProductBaseCode=PS
  MB-PSS  216 : powerlib/Machines/Multi-Band Power System Stabilizer  OperationMode=Simplified settings  Kg=1  GL=[0.1 10]  GI="[1  10]"  GH="[13  120]"  GLd=[66 66 9.4]  TcLF=[1.667 2 0 0 0 0 2 2.4 0 0 0 0 1 1]  GId=[66 66 47.6]  TcIF=[1 1 0.25 0.3 0 0 1 1 0.3 0.36 0 0 0 0]  GHd=[66 66 233]  TcHF="[0.01 0.012 0 0 0 0  0.012 0.0144 0 0 0 0 1 1]"  LIM=[.075 .15 .15 .15]  Plot_On=off  MagdB_On=off  FreqRange=logspace(-2,2,500)
      settings: SourceProductName=Simscape Power Systems  SourceProductBaseCode=PS
  Multiport Switch1 : MultiPortSwitch  Inputs=4  InputSameDT=on
  PSS model3 : Constant  Value=0
  PSS model4 : Constant
  Pref : Constant
  Real-Imag to Complex : RealImagToComplex
  STG 216 : powerlib/Machines/Steam Turbine and Governor  gentype=Tandem-compound (single mass)  reg1="[ 1  0.05    0 ]"  reg2="[ 0.001  0.15 ]"  reg3="[ -0.1  0.1  0  4.496 ]"  N=3600  turb1="[ 0  10   3.3   0.5   ]"  turb2="[   0   0.36    0.36   0.28   ]"  HA="[ 0.046  1.430  1.465   0.192 ]"  KA="[ 90.44  53.88  64.59   62.94  ]"  DA="[ 0.0115  0.3575  0.3663   0.0137  ]"  ini1=0.95  ini2=[0.779316,-31.4247]
      settings: SourceProductName=Simscape Power Systems  SourceProductBaseCode=PS
  Sum2 : Sum  SaturateOnIntegerOverflow=on  InputSameDT=on  OutDataTypeStr=Inherit: Same as first input
  Sum3 : Sum  Inputs=-+  SaturateOnIntegerOverflow=on  InputSameDT=on  OutDataTypeStr=Inherit: Same as first input
  Terminator1 : Terminator
  Terminator2 : Terminator
  Terminator3 : Terminator
  Vref216 : Constant
  wref : Constant
  A : PMIOPort  Side=Left
  B : PMIOPort  Port=2  Side=Left
  C : PMIOPort  Port=3  Side=Left
  tag scope: EFD216=global, Pa216=global, Pe216=global, Pm216=global, Q216=global, Vt216=global, d_theta216=global, pss216=global, theta216=global, w216=global
  wires:
  Bus Selector1/7 -> Real-Imag to Complex/2  "<Stator voltage  vq (pu)>"
  Bus Selector1/6 -> Real-Imag to Complex/1  "<Stator voltage  vd (pu)>"
  wref/1 -> STG 216/1
  Vref216/1 -> AC4A Excitation System 216/1
  Bus Selector1/4 -> [d_theta216], STG 216/4  "<Rotor angle deviation  d_theta (rad)>"
  216/1 -> Bus Selector1/1, [M216]
  Bus Selector1/1 -> [w216], STG 216/3  "<Rotor speed  wm  (pu)>"
  Bus Selector1/3 -> "Delta w PSS (Kundur) 216 "/1, MB-PSS  216/1  "<Rotor speed deviation  dw (pu)>"
  Real-Imag to Complex/1 -> Complex to Magnitude-Angle/1
  Complex to Magnitude-Angle/1 -> AC4A Excitation System 216/2, [Vt216]
  AC4A Excitation System 216/1 -> 216/2, [EFD216]
  Multiport Switch1/1 -> AC4A Excitation System 216/4, [pss216]
  Bus Selector1/5 -> [theta216]  "<Rotor mechanical angle  theta (deg)>"
  Bus Selector1/2 -> [Pe216]  "<Output active power   Peo (pu)>"
  Bus Selector1/8 -> AC4A Excitation System 216/3  "<Field current  ifd (pu)>"
  STG 216/4 -> [Pm216], 216/1
  Pref/1 -> STG 216/2
  Bus Selector1/9 -> [Q216]  "<Output reactive power  Qeo (pu)>"
  PSS model4/1 -> Sum2/2
  Sum2/1 -> Multiport Switch1/1
  [PSSmodel] -> Sum2/1
  PSS model3/1 -> Multiport Switch1/2
  Sum3/1 -> [Pa216], "Delta Pa PSS 216 "/1  "Pm-Pe"
  "Delta Pa PSS 216 "/1 -> Multiport Switch1/5
  "Delta w PSS (Kundur) 216 "/1 -> Multiport Switch1/4
  [Pm216] -> Sum3/2
  [Pe216] -> Sum3/1
  MB-PSS  216/1 -> Multiport Switch1/3
  STG 216/1 -> Terminator3/1
  STG 216/2 -> Terminator1/1
  STG 216/3 -> Terminator2/1
  connections:
  216/RConn1 -- A/RConn1
  216/RConn2 -- B/RConn1
  216/RConn3 -- C/RConn1

== system IEEE24bus/221 ==
  221 : powerlib/Machines/Synchronous Machine pu Standard  PresetModel=No  MechanicalLoad=Mechanical power Pm  ShowDetailedParameters=on  RotorType=Round  Units=per unit standard parameters  MeasurementBus=off  NominalParameters="[190*1E6  G_data(29,3)*1E3  60]"  Reactances1=[G_data(29,6),G_data(29,8),G_data(29,10),G_data(29,7),G_data(29,12),G_data(29,14),G_data(29,5)]  Reactances2=[G_data(6,6),G_data(6,8),G_data(6,10),G_data(6,7),G_data(6,12),G_data(6,14),G_data(6,5)]  dAxisTimeConstants=Open-circuit  qAxisTimeConstants=Open-circuit  TimeConstants1="[G_data(6,9)  G_data(6,11)  G_data(6,13)  G_data(6,15)]"  TimeConstants2="[G_data(29,9)  G_data(29,11)  G_data(29,13)  G_data(29,15)]"  TimeConstants3="[  5.9  0.033  0.023  ]"  TimeConstants4=[ 8.0, 0.03, 0.3371, 0.0295 ]  TimeConstants5=[ 1.01, 0.053, 0.1 ]  TimeConstants6=[ 1.3201, 0.023, 1.0, 0.07 ]  TimeConstants7="[  1.01  0.053  0.051266  ]"  TimeConstants8=[ 1.3201, 0.0231, 0.3371, 0.0295 ]  StatorResistance=0  Mechanical="[ H221 0  4 ]"  PolePairs=4  InitialConditions=[0 -49.0871 0.832503 0.832503 0.832503 -10.6328 -130.633 109.367 2.39024]  SetSaturation=off  Saturation=[0.6404,0.7127,0.8441,0.9214,0.9956,1.082,1.19,1.316,1.457;0.7,0.7698,0.8872,0.9466,0.9969,1.046,1.1,1.151,1.201]  LoadFlowParameters=[1 3330000000 20000 0 0]  TsPowergui=0  TsBlock=-1  IterativeModel=Forward Euler  IterativeDiscreteModel=Trapezoidal non iterative  BusType=PV  Pref=G_data(29,2)*1e6  Qref=0  Qmin=-inf  Qmax=inf  PLF=0  QLF=0
      settings: SourceProductName=Simscape Power Systems
  AC4A Excitation System 221 : sps_avr/AC4A Excitation System  Tr=Exc(29,2)  KaTa="[Exc(29,3)   Exc(29,4)]"  VIminmax=[-10 10]  VRminmax=[-4.53 5.64]  TbTc="[Exc(29,5)  Exc(29,6)]"  Kc=0  v0=[1 2.3902]  TsBlock=0
      settings: SourceProductName=Simscape Power Systems  SourceProductBaseCode=PS
  Bus Selector1 : BusSelector  OutputSignals="Mechanical.Rotor speed  wm  (pu),Output active power   Peo (pu),Mechanical.Rotor speed deviation  dw (pu),Mechanical.Rotor angle deviation  d_theta (rad),Mechanical.Rotor mechanical angle  theta (deg),dq0 components.Stator voltage  vd (pu),dq0 components.Stator voltage  vq (pu),dq0 components.Field current  ifd (pu),Output reactive power  Qeo (pu)"
  Complex to Magnitude-Angle : ComplexToMagnitudeAngle  Output=Magnitude
  "Delta Pa PSS 221 " : powerlib/Machines/Generic Power System Stabilizer  Tsensor=15e-3  K=2.5*1.25  Twashout=1  Tleadlag1=[60e-3 1]  Tleadlag2=[0 0]  VSlimits=[-0.15 0.15]  Vinit=0  Plot_On=off  MagdB_On=on  FreqRange=logspace(-2,2,500)
      settings: SourceProductName=Simscape Power Systems  SourceProductBaseCode=PS
  Delta w PSS (Kundur) 221 : powerlib/Machines/Generic Power System Stabilizer  Tsensor=15e-3  K=30  Twashout=10  Tleadlag1=[50e-3 20e-3]  Tleadlag2=[3 5.4]  VSlimits=[-0.15 0.15]  Vinit=0  Plot_On=off  MagdB_On=on  FreqRange=logspace(-2,2,500)
      settings: SourceProductName=Simscape Power Systems  SourceProductBaseCode=PS
  MB-PSS  221 : powerlib/Machines/Multi-Band Power System Stabilizer  OperationMode=Simplified settings  Kg=1  GL=[0.1 10]  GI="[1  10]"  GH="[13  120]"  GLd=[66 66 9.4]  TcLF=[1.667 2 0 0 0 0 2 2.4 0 0 0 0 1 1]  GId=[66 66 47.6]  TcIF=[1 1 0.25 0.3 0 0 1 1 0.3 0.36 0 0 0 0]  GHd=[66 66 233]  TcHF="[0.01 0.012 0 0 0 0  0.012 0.0144 0 0 0 0 1 1]"  LIM=[.075 .15 .15 .15]  Plot_On=off  MagdB_On=off  FreqRange=logspace(-2,2,500)
      settings: SourceProductName=Simscape Power Systems  SourceProductBaseCode=PS
  Multiport Switch1 : MultiPortSwitch  Inputs=4  InputSameDT=on
  PSS model3 : Constant  Value=0
  PSS model4 : Constant
  Pref : Constant
  Real-Imag to Complex : RealImagToComplex
  STG 221 : powerlib/Machines/Steam Turbine and Governor  gentype=Tandem-compound (single mass)  reg1="[ 1  0.05    0 ]"  reg2="[ 0.001  0.15 ]"  reg3="[ -0.1  0.1  0  4.496 ]"  N=3600  turb1="[ 0  10   3.3   0.5   ]"  turb2="[   0   0.36    0.36   0.28   ]"  HA="[ 0.046  1.430  1.465   0.192 ]"  KA="[ 90.44  53.88  64.59   62.94  ]"  DA="[ 0.0115  0.3575  0.3663   0.0137  ]"  ini1=1  ini2=[0.779316,-31.4247]
      settings: SourceProductName=Simscape Power Systems  SourceProductBaseCode=PS
  Sum2 : Sum  SaturateOnIntegerOverflow=on  InputSameDT=on  OutDataTypeStr=Inherit: Same as first input
  Sum3 : Sum  Inputs=-+  SaturateOnIntegerOverflow=on  InputSameDT=on  OutDataTypeStr=Inherit: Same as first input
  Terminator1 : Terminator
  Terminator2 : Terminator
  Terminator3 : Terminator
  Vref22 : Constant
  wref : Constant
  A : PMIOPort  Side=Left
  B : PMIOPort  Port=2  Side=Left
  C : PMIOPort  Port=3  Side=Left
  tag scope: EFD221=global, Pa221=global, Pe221=global, Pm221=global, Q221=global, Vt221=global, d_theta221=global, pss221=global, theta221=global, w221=global
  wires:
  Bus Selector1/7 -> Real-Imag to Complex/2  "<Stator voltage  vq (pu)>"
  Bus Selector1/6 -> Real-Imag to Complex/1  "<Stator voltage  vd (pu)>"
  wref/1 -> STG 221/1
  Vref22/1 -> AC4A Excitation System 221/1
  Bus Selector1/4 -> [d_theta221], STG 221/4  "<Rotor angle deviation  d_theta (rad)>"
  221/1 -> Bus Selector1/1, [M221]
  Bus Selector1/1 -> [w221], STG 221/3  "<Rotor speed  wm  (pu)>"
  Bus Selector1/3 -> Delta w PSS (Kundur) 221/1, MB-PSS  221/1  "<Rotor speed deviation  dw (pu)>"
  Real-Imag to Complex/1 -> Complex to Magnitude-Angle/1
  Complex to Magnitude-Angle/1 -> AC4A Excitation System 221/2, [Vt221]
  AC4A Excitation System 221/1 -> 221/2, [EFD221]
  Multiport Switch1/1 -> AC4A Excitation System 221/4, [pss221]
  Bus Selector1/5 -> [theta221]  "<Rotor mechanical angle  theta (deg)>"
  Bus Selector1/2 -> [Pe221]  "<Output active power   Peo (pu)>"
  Bus Selector1/8 -> AC4A Excitation System 221/3  "<Field current  ifd (pu)>"
  STG 221/4 -> [Pm221], 221/1
  Pref/1 -> STG 221/2
  Bus Selector1/9 -> [Q221]  "<Output reactive power  Qeo (pu)>"
  PSS model4/1 -> Sum2/2
  Sum2/1 -> Multiport Switch1/1
  [PSSmodel] -> Sum2/1
  PSS model3/1 -> Multiport Switch1/2
  Sum3/1 -> [Pa221], "Delta Pa PSS 221 "/1  "Pm-Pe"
  "Delta Pa PSS 221 "/1 -> Multiport Switch1/5
  Delta w PSS (Kundur) 221/1 -> Multiport Switch1/4
  [Pm221] -> Sum3/2
  [Pe221] -> Sum3/1
  MB-PSS  221/1 -> Multiport Switch1/3
  STG 221/1 -> Terminator3/1
  STG 221/2 -> Terminator1/1
  STG 221/3 -> Terminator2/1
  connections:
  221/RConn1 -- A/RConn1
  221/RConn2 -- B/RConn1
  221/RConn3 -- C/RConn1

== system IEEE24bus/231 ==
  231 : powerlib/Machines/Synchronous Machine pu Standard  PresetModel=No  MechanicalLoad=Mechanical power Pm  ShowDetailedParameters=on  RotorType=Round  Units=per unit standard parameters  MeasurementBus=off  NominalParameters="[210*1E6  G_data(30,3)*1E3  60]"  Reactances1=[G_data(30,6),G_data(10,8),G_data(30,10),G_data(30,7),G_data(30,12),G_data(30,14),G_data(30,5)]  Reactances2=[G_data(6,6),G_data(6,8),G_data(6,10),G_data(6,7),G_data(6,12),G_data(6,14),G_data(6,5)]  dAxisTimeConstants=Open-circuit  qAxisTimeConstants=Open-circuit  TimeConstants1="[G_data(6,9)  G_data(6,11)  G_data(6,13)  G_data(6,15)]"  TimeConstants2="[G_data(30,9)  G_data(30,11)  G_data(30,13)  G_data(30,15)]"  TimeConstants3="[  5.9  0.033  0.023  ]"  TimeConstants4=[ 8.0, 0.03, 0.3371, 0.0295 ]  TimeConstants5=[ 1.01, 0.053, 0.1 ]  TimeConstants6=[ 1.3201, 0.023, 1.0, 0.07 ]  TimeConstants7="[  1.01  0.053  0.051266  ]"  TimeConstants8=[ 1.3201, 0.0231, 0.3371, 0.0295 ]  StatorResistance=0  Mechanical="[ H231 0  4 ]"  PolePairs=4  InitialConditions=[0 -49.0871 0.832503 0.832503 0.832503 -10.6328 -130.633 109.367 2.39024]  SetSaturation=off  Saturation=[0.6404,0.7127,0.8441,0.9214,0.9956,1.082,1.19,1.316,1.457;0.7,0.7698,0.8872,0.9466,0.9969,1.046,1.1,1.151,1.201]  LoadFlowParameters=[1 3330000000 20000 0 0]  TsPowergui=0  TsBlock=-1  IterativeModel=Forward Euler  IterativeDiscreteModel=Trapezoidal non iterative  BusType=PV  Pref=210*1e6  Qref=0  Qmin=-inf  Qmax=inf  PLF=0  QLF=0
      settings: SourceProductName=Simscape Power Systems
  AC4A Excitation System 231 : sps_avr/AC4A Excitation System  Tr=Exc(30,2)  KaTa="[Exc(30,3)   Exc(30,4)]"  VIminmax=[-10 10]  VRminmax=[-4.53 5.64]  TbTc="[Exc(30,5)  Exc(30,6)]"  Kc=0  v0=[1 2.3902]  TsBlock=0
      settings: SourceProductName=Simscape Power Systems  SourceProductBaseCode=PS
  Bus Selector1 : BusSelector  OutputSignals="Mechanical.Rotor speed  wm  (pu),Output active power   Peo (pu),Mechanical.Rotor speed deviation  dw (pu),Mechanical.Rotor angle deviation  d_theta (rad),Mechanical.Rotor mechanical angle  theta (deg),dq0 components.Stator voltage  vd (pu),dq0 components.Stator voltage  vq (pu),dq0 components.Field current  ifd (pu),Output reactive power  Qeo (pu)"
  Complex to Magnitude-Angle : ComplexToMagnitudeAngle  Output=Magnitude
  "Delta Pa PSS 231 " : powerlib/Machines/Generic Power System Stabilizer  Tsensor=15e-3  K=2.5*1.25  Twashout=1  Tleadlag1=[60e-3 1]  Tleadlag2=[0 0]  VSlimits=[-0.15 0.15]  Vinit=0  Plot_On=off  MagdB_On=on  FreqRange=logspace(-2,2,500)
      settings: SourceProductName=Simscape Power Systems  SourceProductBaseCode=PS
  "Delta w PSS (Kundur) 231 " : powerlib/Machines/Generic Power System Stabilizer  Tsensor=15e-3  K=30  Twashout=10  Tleadlag1=[50e-3 20e-3]  Tleadlag2=[3 5.4]  VSlimits=[-0.15 0.15]  Vinit=0  Plot_On=off  MagdB_On=on  FreqRange=logspace(-2,2,500)
      settings: SourceProductName=Simscape Power Systems  SourceProductBaseCode=PS
  MB-PSS  231 : powerlib/Machines/Multi-Band Power System Stabilizer  OperationMode=Simplified settings  Kg=1  GL=[0.1 10]  GI="[1  10]"  GH="[13  120]"  GLd=[66 66 9.4]  TcLF=[1.667 2 0 0 0 0 2 2.4 0 0 0 0 1 1]  GId=[66 66 47.6]  TcIF=[1 1 0.25 0.3 0 0 1 1 0.3 0.36 0 0 0 0]  GHd=[66 66 233]  TcHF="[0.01 0.012 0 0 0 0  0.012 0.0144 0 0 0 0 1 1]"  LIM=[.075 .15 .15 .15]  Plot_On=off  MagdB_On=off  FreqRange=logspace(-2,2,500)
      settings: SourceProductName=Simscape Power Systems  SourceProductBaseCode=PS
  Multiport Switch1 : MultiPortSwitch  Inputs=4  InputSameDT=on
  PSS model3 : Constant  Value=0
  PSS model4 : Constant
  Pref : Constant
  Real-Imag to Complex : RealImagToComplex
  STG 231 : powerlib/Machines/Steam Turbine and Governor  gentype=Tandem-compound (single mass)  reg1="[ 1  0.05    0 ]"  reg2="[ 0.001  0.15 ]"  reg3="[ -0.1  0.1  0  4.496 ]"  N=3600  turb1="[ 0  10   3.3   0.5   ]"  turb2="[   0   0.36    0.36   0.28   ]"  HA="[ 0.046  1.430  1.465   0.192 ]"  KA="[ 90.44  53.88  64.59   62.94  ]"  DA="[ 0.0115  0.3575  0.3663   0.0137  ]"  ini1=0.99  ini2=[0.779316,-31.4247]
      settings: SourceProductName=Simscape Power Systems  SourceProductBaseCode=PS
  Sum2 : Sum  SaturateOnIntegerOverflow=on  InputSameDT=on  OutDataTypeStr=Inherit: Same as first input
  Sum3 : Sum  Inputs=-+  SaturateOnIntegerOverflow=on  InputSameDT=on  OutDataTypeStr=Inherit: Same as first input
  Terminator1 : Terminator
  Terminator2 : Terminator
  Terminator3 : Terminator
  Vref23 : Constant
  wref : Constant
  A : PMIOPort  Side=Left
  B : PMIOPort  Port=2  Side=Left
  C : PMIOPort  Port=3  Side=Left
  tag scope: EFD231=global, Pa231=global, Pe231=global, Pm231=global, Q231=global, Vt231=global, d_theta231=global, pss231=global, theta231=global, w231=global
  wires:
  Bus Selector1/7 -> Real-Imag to Complex/2  "<Stator voltage  vq (pu)>"
  Bus Selector1/6 -> Real-Imag to Complex/1  "<Stator voltage  vd (pu)>"
  wref/1 -> STG 231/1
  Vref23/1 -> AC4A Excitation System 231/1
  Bus Selector1/4 -> [d_theta231], STG 231/4  "<Rotor angle deviation  d_theta (rad)>"
  231/1 -> Bus Selector1/1, [M231]
  Bus Selector1/1 -> [w231], STG 231/3  "<Rotor speed  wm  (pu)>"
  Bus Selector1/3 -> "Delta w PSS (Kundur) 231 "/1, MB-PSS  231/1  "<Rotor speed deviation  dw (pu)>"
  Real-Imag to Complex/1 -> Complex to Magnitude-Angle/1
  Complex to Magnitude-Angle/1 -> AC4A Excitation System 231/2, [Vt231]
  AC4A Excitation System 231/1 -> 231/2, [EFD231]
  Multiport Switch1/1 -> AC4A Excitation System 231/4, [pss231]
  Bus Selector1/5 -> [theta231]  "<Rotor mechanical angle  theta (deg)>"
  Bus Selector1/2 -> [Pe231]  "<Output active power   Peo (pu)>"
  Bus Selector1/8 -> AC4A Excitation System 231/3  "<Field current  ifd (pu)>"
  STG 231/4 -> [Pm231], 231/1
  Pref/1 -> STG 231/2
  Bus Selector1/9 -> [Q231]  "<Output reactive power  Qeo (pu)>"
  PSS model4/1 -> Sum2/2
  Sum2/1 -> Multiport Switch1/1
  [PSSmodel] -> Sum2/1
  PSS model3/1 -> Multiport Switch1/2
  Sum3/1 -> [Pa231], "Delta Pa PSS 231 "/1  "Pm-Pe"
  "Delta Pa PSS 231 "/1 -> Multiport Switch1/5
  "Delta w PSS (Kundur) 231 "/1 -> Multiport Switch1/4
  [Pm231] -> Sum3/2
  [Pe231] -> Sum3/1
  MB-PSS  231/1 -> Multiport Switch1/3
  STG 231/1 -> Terminator3/1
  STG 231/2 -> Terminator1/1
  STG 231/3 -> Terminator2/1
  connections:
  231/RConn1 -- A/RConn1
  231/RConn2 -- B/RConn1
  231/RConn3 -- C/RConn1
